simulink model "EE405L_Lab2_E2"  (R2021b)
settings: Solver=VariableStepAuto  StartTime=0.0  StopTime=10.0  RelTol=1e-3
settings Model: Creator=Kevin  LastModifiedBy=Kevin

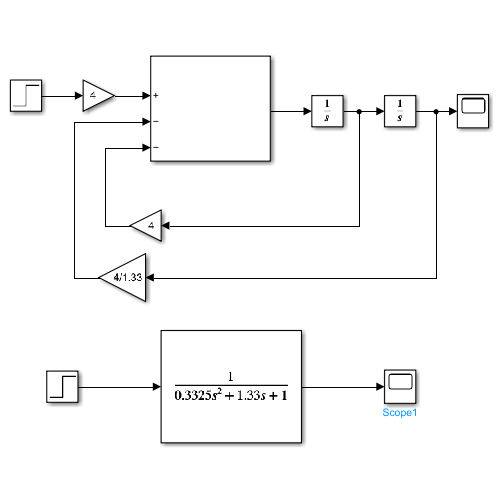
[thumbnail: Simulink's stored preview of the top-level diagram]
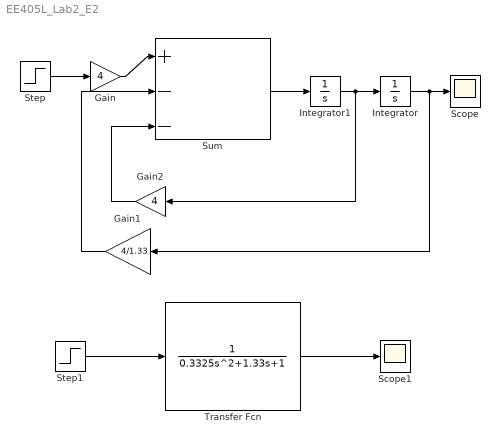
== system EE405L_Lab2_E2 ==
  Gain : Gain  Gain=4
  Gain1 : Gain  Gain=4/1.33
  Gain2 : Gain  Gain=4
  Integrator : Integrator
  Integrator1 : Integrator
  Scope : Scope
  Scope1 : Scope
  Step : Step  SampleTime=0
  Step1 : Step  SampleTime=0
  Sum : Sum  Inputs=|+--
  Transfer Fcn : TransferFcn  Denominator=[0.3325 1.33 1]
  wires:
  Step/1 -> Gain/1
  Gain/1 -> Sum/1
  Gain2/1 -> Sum/3
  Gain1/1 -> Sum/2
  Sum/1 -> Integrator1/1
  Integrator1/1 -> Gain2/1, Integrator/1
  Integrator/1 -> Gain1/1, Scope/1
  Step1/1 -> Transfer Fcn/1
  Transfer Fcn/1 -> Scope1/1
